simulink model "T6_Q5_sim"  (R2023b)
settings: Solver=VariableStepAuto  StartTime=0.0  StopTime=100  FixedStep=0.01  MaxStep=0.001  RelTol=1e-6
settings Model: Creator=truel  LastModifiedBy=truel

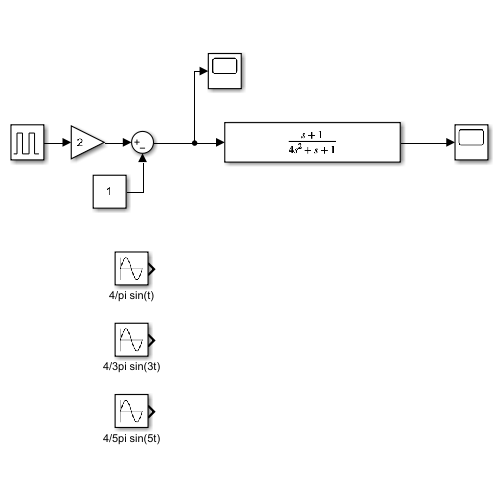
[thumbnail: Simulink's stored preview of the top-level diagram]
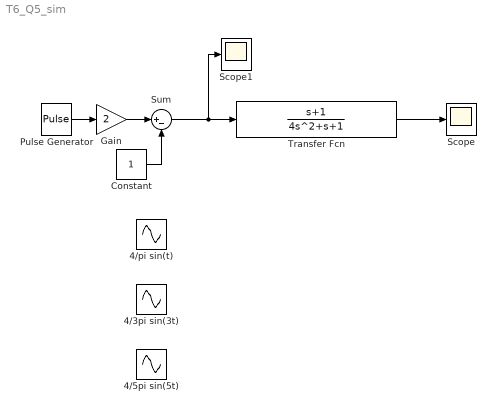
== system T6_Q5_sim ==
  4/3pi sin(3t) : Sin  Amplitude=4/pi*1/3  Frequency=3  SampleTime=0
  4/5pi sin(5t) : Sin  Amplitude=4/pi*1/5  Frequency=5  SampleTime=0
  4/pi sin(t) : Sin  Amplitude=4/pi  SampleTime=0
  Constant : Constant
  Gain : Gain  Gain=2
  Pulse Generator : DiscretePulseGenerator  PulseType=Time based  Period=2*pi  PulseWidth=50
  Scope : Scope
  Scope1 : Scope
  Sum : Sum  Inputs=|+-
  Transfer Fcn : TransferFcn  Numerator=[1 1]  Denominator=[4 1 1]
  wires:
  Pulse Generator/1 -> Gain/1
  Transfer Fcn/1 -> Scope/1
  Gain/1 -> Sum/1
  Constant/1 -> Sum/2
  Sum/1 -> Scope1/1, Transfer Fcn/1
